simulink model "CTS_State_Estimator_Fault"  (R2023a)
settings: Solver=VariableStepAuto  StartTime=0.0  StopTime=10.0  RelTol=1e-3
undefined symbols (not defined in the file): A, A_1, A_2, B, C, c_1, c_2, G, h_10, h_20, ICs, q_i, q_i0
settings Model: Creator=m260477  LastModifiedBy=m260477
settings DataIOCC: Refine=5

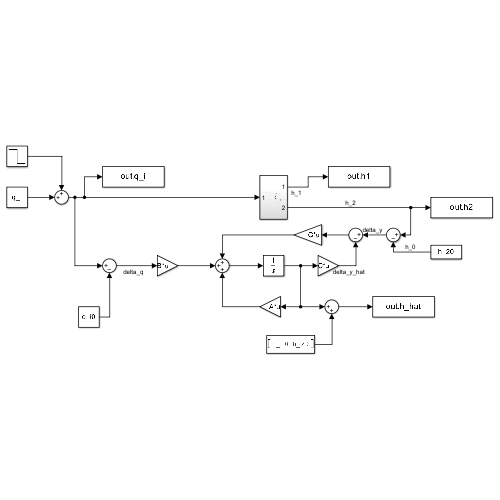
[thumbnail: Simulink's stored preview of the top-level diagram]
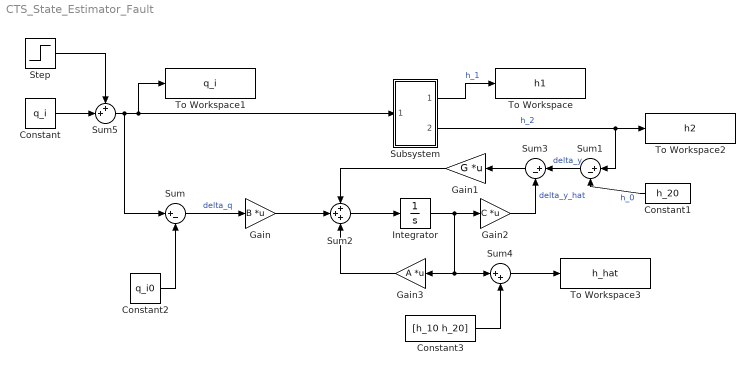
== system CTS_State_Estimator_Fault ==
  Constant : Constant  Value=q_i
  Constant1 : Constant  Value=h_20
  Constant2 : Constant  Value=q_i0
  Constant3 : Constant  Value=[h_10 h_20]
  Gain : Gain  Gain=B  Multiplication=Matrix(K*u)
  Gain1 : Gain  Gain=G  Multiplication=Matrix(K*u)
  Gain2 : Gain  Gain=C  Multiplication=Matrix(K*u)
  Gain3 : Gain  Gain=A  Multiplication=Matrix(K*u)
  Integrator : Integrator  InitialCondition=ICs
  Step : Step  Time=100  After=-0.5*q_i  SampleTime=0
  Subsystem : Subsystem
  Sum : Sum  Inputs=|+-
  Sum1 : Sum  Inputs=|+-
  Sum2 : Sum  Inputs=+++
  Sum3 : Sum  Inputs=|+-
  Sum4 : Sum  Inputs=|++
  Sum5 : Sum  Inputs=++|
  To Workspace : ToWorkspace  VariableName=h1  SaveFormat=Timeseries  SampleTime=-1
  To Workspace1 : ToWorkspace  VariableName=q_i  SaveFormat=Timeseries  SampleTime=-1
  To Workspace2 : ToWorkspace  VariableName=h2  SaveFormat=Timeseries  SampleTime=-1
  To Workspace3 : ToWorkspace  VariableName=h_hat  SaveFormat=Timeseries  SampleTime=-1
  wires:
  Subsystem/2(Out3) -> Sum1/1, To Workspace2/1  "h_2"
  Constant2/1 -> Sum/2
  Constant1/1 -> Sum1/2  "h_0"
  Sum/1 -> Gain/1  "delta_q"
  Gain1/1 -> Sum2/1
  Gain/1 -> Sum2/2
  Sum2/1 -> Integrator/1
  Integrator/1 -> Sum4/1, Gain3/1, Gain2/1
  Gain2/1 -> Sum3/2  "delta_y_hat"
  Sum1/1 -> Sum3/1  "delta_y"
  Sum3/1 -> Gain1/1
  Gain3/1 -> Sum2/3
  Subsystem/1(Out1) -> To Workspace/1  "h_1"
  Constant3/1 -> Sum4/2
  Sum4/1 -> To Workspace3/1
  Constant/1 -> Sum5/2
  Sum5/1 -> Sum/1, To Workspace1/1, Subsystem/1(Input)
  Step/1 -> Sum5/1

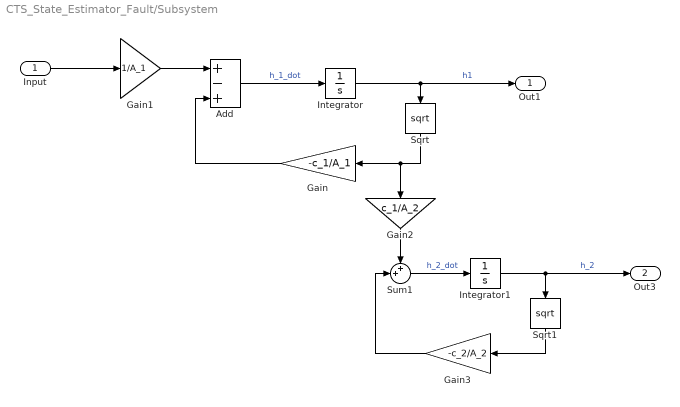
== system CTS_State_Estimator_Fault/Subsystem ==
  Input : Inport
  Add : Sum  Inputs=+-+
  Gain : Gain  Gain=-c_1/A_1
  Gain1 : Gain  Gain=1/A_1
  Gain2 : Gain  Gain=c_1/A_2
  Gain3 : Gain  Gain=-c_2/A_2
  Integrator : Integrator  InitialCondition=ICs
  Integrator1 : Integrator  InitialCondition=ICs
  Sqrt : Sqrt
  Sqrt1 : Sqrt
  Sum1 : Sum  Inputs=++|
  Out1 : Outport
  Out3 : Outport  Port=2
  wires:
  Integrator1/1 -> Out3/1, Sqrt1/1  "h_2"
  Input/1 -> Gain1/1
  Gain1/1 -> Add/1
  Sqrt1/1 -> Gain3/1
  Gain2/1 -> Sum1/1
  Integrator/1 -> Out1/1, Sqrt/1  "h1"
  Add/1 -> Integrator/1  "h_1_dot"
  Gain3/1 -> Sum1/2
  Sum1/1 -> Integrator1/1  "h_2_dot"
  Gain/1 -> Add/3
  Sqrt/1 -> Gain2/1, Gain/1
